simulink model "c250_bb2"  (R2012b)
(part 2 of 39)

  FIR1/1(data_out) -> Delay28/1
  FIR2/1(data_out) -> Delay34/1
  FIR2/2(ch_out) -> Delay35/1
  FIR3/1(data_out) -> Delay36/1
  FIR3/2(ch_out) -> Delay37/1
  mixer1/1(data_out) -> conv_phase1/1(data_in), Delay24/1
  accumulator1/1(data_out) -> avgIQ1/1(din)
  accumulator1/2(drdy) -> avgIQ1/3(we)
  Delay24/1 -> Delay23/1
  Relational2/1 -> Logical1/1
  Constant4/1 -> Relational2/2
  Logical1/1 -> pulse_ext1/1
  pulse_ext1/1 -> accumulator1/2(accum_en)
  Delay23/1 -> Delay25/1
  Delay25/1 -> accumulator1/1(data_in)
  mixer2/1(data_out) -> conv_phase2/1(data_in), Delay29/1
  accumulator2/1(data_out) -> avgIQ2/1(din)
  accumulator2/2(drdy) -> avgIQ2/3(we)
  Delay29/1 -> Delay27/1
  Relational3/1 -> Logical2/1
  Constant15/1 -> Relational3/2
  Logical2/1 -> pulse_ext3/1
  pulse_ext3/1 -> accumulator2/2(accum_en)
  Delay27/1 -> Delay32/1
  Delay32/1 -> accumulator2/1(data_in)
  mixer3/1(data_out) -> conv_phase3/1(data_in), Delay41/1
  accumulator3/1(data_out) -> avgIQ3/1(din)
  accumulator3/2(drdy) -> avgIQ3/3(we)
  Delay41/1 -> Delay33/1
  Relational4/1 -> Logical3/1
  Constant17/1 -> Relational4/2
  Logical3/1 -> pulse_ext6/1
  pulse_ext6/1 -> accumulator3/2(accum_en)
  Slice2/1 -> avgIQ/2(trig), avgIQ1/2(trig), avgIQ3/2(trig), avgIQ2/2(trig), posedge/1(in)
  Delay33/1 -> Delay48/1
  Delay48/1 -> accumulator3/1(data_in)
  Delay49/1 -> conv_phase2/2(ch_in), Relational3/1, conv_phase1/2(ch_in), Relational2/1, Relational1/1, conv_phase0/2(ch_in), conv_phase3/2(ch_in), Relational4/1
  capture1/1(data_out) -> Delay50/1
  capture1/2(we_out) -> Delay52/1
  capture1/3(sync_out) -> Delay73/1
  capture2/1(data_out) -> Delay74/1
  capture2/2(we_out) -> Delay75/1
  capture2/3(sync_out) -> Delay76/1
  capture3/1(data_out) -> Delay77/1
  capture3/2(we_out) -> Delay78/1
  capture3/3(sync_out) -> Delay79/1
  bins17/1(in_reg) -> Slice1/1
  Slice1/1 -> [dds_I0]
  bins1/1(in_reg) -> Slice6/1
  Slice6/1 -> [dds_Q0]
  bins2/1(in_reg) -> Slice7/1
  Slice7/1 -> [dds_I1]
  bins3/1(in_reg) -> Slice8/1
  Slice8/1 -> [dds_Q1]
  bins4/1(in_reg) -> Slice9/1
  Slice9/1 -> PFB/1
  bins5/1(in_reg) -> Slice10/1
  Slice10/1 -> PFB/2
  bins6/1(in_reg) -> Slice13/1
  Slice13/1 -> PFB/3
  bins7/1(in_reg) -> Slice14/1
  Slice14/1 -> PFB/4
  bins8/1(in_reg) -> Slice15/1
  Slice15/1 -> PFB/5
  bins9/1(in_reg) -> Slice17/1
  Slice17/1 -> PFB/6
  bins10/1(in_reg) -> Slice19/1
  Slice19/1 -> PFB/7
  bins11/1(in_reg) -> Slice21/1
  Slice21/1 -> PFB/8
  bins12/1(in_reg) -> Slice26/1
  Slice26/1 -> PFB/9
  bins13/1(in_reg) -> Slice27/1
  Slice27/1 -> PFB/10
  bins14/1(in_reg) -> Slice28/1
  Slice28/1 -> PFB/11
  bins15/1(in_reg) -> Slice29/1
  Slice29/1 -> PFB/12
  bins16/1(in_reg) -> Slice30/1
  Slice30/1 -> PFB/13
  bins18/1(in_reg) -> Slice31/1
  Slice31/1 -> PFB/14
  bins19/1(in_reg) -> Slice32/1
  Slice32/1 -> PFB/15
  bins20/1(in_reg) -> Slice33/1
  Slice33/1 -> PFB/16
  Delay21/1 -> capture/1(data_in)
  Delay22/1 -> capture/2(ch_in)
  Delay28/1 -> capture1/1(data_in)
  Delay31/1 -> capture1/2(ch_in)
  Delay34/1 -> capture2/1(data_in)
  Delay35/1 -> capture2/2(ch_in)
  Delay36/1 -> capture3/1(data_in)
  Delay37/1 -> capture3/2(ch_in)
  Delay46/1 -> Logical5/1, LUT Counter2/2
  Delay50/1 -> Terminator1/1
  Delay52/1 -> Terminator2/1
  Delay73/1 -> Terminator3/1
  Delay74/1 -> Terminator4/1
  Delay75/1 -> Terminator6/1
  Delay76/1 -> Terminator7/1
  Delay77/1 -> Terminator8/1
  Delay78/1 -> Terminator9/1
  Delay79/1 -> Terminator10/1
  Slice34/1 -> Delay54/1
  Delay55/1 -> mixer1/1(data_in)
  Delay56/1 -> mixer2/1(data_in)
  Delay57/1 -> mixer3/1(data_in)
  Delay59/1 -> Delay49/1
  BitBasher/1 -> mixer0/2(dds_I0)
  BitBasher/2 -> mixer0/3(dds_Q0)
  BitBasher/3 -> mixer0/4(dds_I1)
  BitBasher/4 -> mixer0/5(dds_Q1)
  BitBasher1/1 -> mixer1/2(dds_I0)
  BitBasher1/2 -> mixer1/3(dds_Q0)
  BitBasher1/3 -> mixer1/4(dds_I1)
  BitBasher1/4 -> mixer1/5(dds_Q1)
  BitBasher2/1 -> mixer2/2(dds_I0)
  BitBasher2/2 -> mixer2/3(dds_Q0)
  BitBasher2/3 -> mixer2/4(dds_I1)
  BitBasher2/4 -> mixer2/5(dds_Q1)
  BitBasher3/1 -> mixer3/2(dds_I0)
  BitBasher3/2 -> mixer3/3(dds_Q0)
  BitBasher3/3 -> mixer3/4(dds_I1)
  BitBasher3/4 -> mixer3/5(dds_Q1)
  dds_lut/1(dds0) -> BitBasher/1
  dds_lut/2(dds1) -> BitBasher1/1
  dds_lut/3(dds2) -> BitBasher2/1
  dds_lut/4(dds3) -> BitBasher3/1
  Delay43/1 -> Terminator11/1
  Delay44/1 -> Terminator12/1
  Register/1 -> Terminator13/1
  Convert/1 -> LUT Counter/1, Delay71/1
